simulink model "Senorless"  (R2023a)
settings: Solver=FixedStepDiscrete  StartTime=0.0  StopTime=5  FixedStep=1/FOC_FRQ  RelTol=1e-3
values from neighbouring files (symbols this model uses):
  ADC_REF = 3.6    [Senorless.sldd]
  ADC_SAMPLE_MAX = 32767.0    [Senorless.sldd]
  AMP_GAIN = 16.0    [Senorless.sldd]
  CURR_INPUT = 3276.0    [Senorless.sldd]
  CURR_KI = 380.0    [Senorless.sldd]
  CURR_KP = 0.04    [Senorless.sldd]
  CURR_LIMIT = 0.95    [Senorless.sldd]
  CURR_OVER = 6.0    [Senorless.sldd]
  CURR_POINT_GAIN = 7.0    [Senorless.sldd]
  CURR_STEP = 32760.0    [Senorless.sldd]
  CURR_UNDER = 0.03    [Senorless.sldd]
  CURR_WIDTH = 6552.0    [Senorless.sldd]
  FOC_FRQ = 25000.0    [Senorless.sldd]
  GAMMA = 32767.0    [Senorless.sldd]
  IMAX = 10.0    [Senorless.sldd]
  LPF_FRQ = 2000.0    [Senorless.sldd]
  MOTOR_DAMPER = 2.06E-7    [Senorless.sldd]
  MOTOR_FLUX = 0.00212352    [Senorless.sldd]
  MOTOR_INERTIA = 4.0E-7    [Senorless.sldd]
  MOTOR_LS = 0.000536    [Senorless.sldd]
  MOTOR_PN = 7.0    [Senorless.sldd]
  MOTOR_RS = 4.0    [Senorless.sldd]
  OPEN_IQ = 0.28    [Senorless.sldd]
  OPEN_IQ_MIN = 0.05    [Senorless.sldd]
  OPEN_IQ_SLOW = 0.1    [Senorless.sldd]
  OPEN_SPD = 1000.0    [Senorless.sldd]
  OPEN_SPD_SLOW = 180.0    [Senorless.sldd]
  OPEN_TIME = 0.5    [Senorless.sldd]
  OPEN_TIME_NFO = 0.5    [Senorless.sldd]
  PLL_LIMIT = 0.9    [Senorless.sldd]
  PLL_WIDTH = 800.0    [Senorless.sldd]
  PWM_FRQ = 96000000.0    [Senorless.sldd]
  RS_HUNT = 0.02    [Senorless.sldd]
  SMOK_FRQ = 600.0    [Senorless.sldd]
  SPD_LIMIT = 0.9    [Senorless.sldd]
  SPD_LPF_LEVEL = 0.0    [Senorless.sldd]
  SPD_MAX = 12000.0    [Senorless.sldd]
  SPD_MIN = 4000.0    [Senorless.sldd]
  SPD_REDUCE = 380.0    [Senorless.sldd]
  SPD_STEP = 6.0    [Senorless.sldd]
  SPD_WIDTH = 20.0    [Senorless.sldd]
  THETA_ERR_LIMIT = 8192.0    [Senorless.sldd]
  TS_POINT_GAIN = 10.0    [Senorless.sldd]
  UDC = 48.0    [Senorless.sldd]
  UDC_GAIN = 21.0    [Senorless.sldd]
  UDC_POINT_GAIN = 10.0    [Senorless.sldd]
undefined symbols (not defined in the file or in its folder): curr_q_ki, curr_q_kp, DiscIntNeverNeededParam, magnitude, PLL_LPF_LEVEL, Udc
libraries: simulink x20, slpidlib x5, mcbcontrolslib x2, mcbplantlib x1, autolibpmsmexterior x1, spspowerguiLib x1
(part 1 of 8)
settings Model: DataDictionary=Senorless.sldd  NumberOfSteps=100  SnapshotBufferSize=5000  SnapshotInterval=5000  Creator=lzm  LastModifiedBy=liangzhuoming
settings DataIOCC: ReturnWorkspaceOutputs=off
settings OptimizationCC: DefaultParameterBehavior=Inlined  GainParamInheritBuiltInType=on  UseFloatMulNetSlope=on  InheritOutputTypeSmallerThanSingle=on  DefaultUnderspecifiedDataType=single  UseSpecifiedMinMax=on  InlineInvariantSignals=on  PassReuseOutputArgsAs=Individual arguments  ZeroExternalMemoryAtStartup=off  ZeroInternalMemoryAtStartup=off  NoFixptDivByZeroProtection=on  EfficientFloat2IntCast=on  LifeSpan=1  OptimizeBlockOrder=speed  DifferentSizesBufferReuse=on  EfficientTunableParamExpr=on
settings DebuggingCC: SignalRangeChecking=warning  ParameterTunabilityLossMsg=error  UnconnectedInputMsg=warning  UnconnectedOutputMsg=warning  UnconnectedLineMsg=warning
settings HardwareCC: ProdBitPerPointer=32  ProdBitPerSizeT=32  ProdBitPerPtrDiffT=32  ProdLargestAtomicInteger=Long  ProdLargestAtomicFloat=Double  ProdWordSize=32  ProdLongLongMode=on  ProdHWDeviceType=ARM Compatible->ARM Cortex-M
settings ModelReferenceCC: EnableRefExpFcnMdlSchedulingChecks=on
settings SFSimCC: MATLABDynamicMemAlloc=off
settings RTWCC: Description=Embedded Coder  SystemTargetFile=ert.tlc  GenCodeOnly=on  TemplateMakefile=ert_default_tmf  GenerateReport=on  BuildConfiguration=Faster Runs  LaunchReport=on  GenerateCodeReplacementReport=on  DLArmComputeVersion=19.05
settings CodeAppCC: ForceParamTrailComments=on  IgnoreCustomStorageClasses=off  OperatorAnnotations=on  SimulinkDataObjDesc=on  SFDataObjDesc=on  CustomSymbolStrGlobalVar=rt$N$M  CustomSymbolStrType=$N$M  CustomSymbolStrFcn=$N$M$F  CustomSymbolStrMacro=$N$M  InsertBlockDesc=on
settings ERTTargetCC: TargetLangStandard=C99 (ISO)  GenerateSampleERTMain=on  IncludeMdlTerminateFcn=off  CombineSignalStateStructs=on  SupportNonFinite=off  SupportComplex=off  SupportNonInlinedSFcns=on  InlinedParameterPlacement=NonHierarchical  ERTCustomFileTemplate=example_file_process.tlc  ERTFilePackagingFormat=CompactWithDataFile

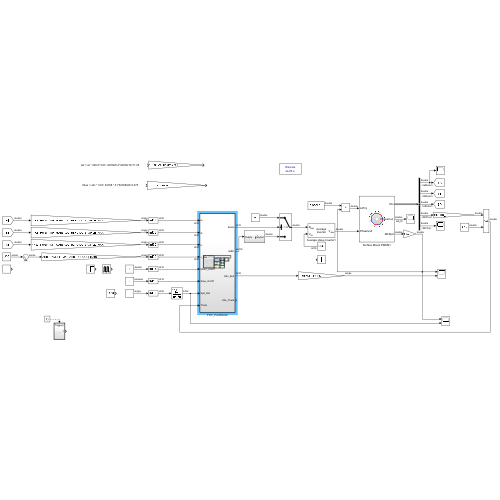
[thumbnail: Simulink's stored preview of the top-level diagram]
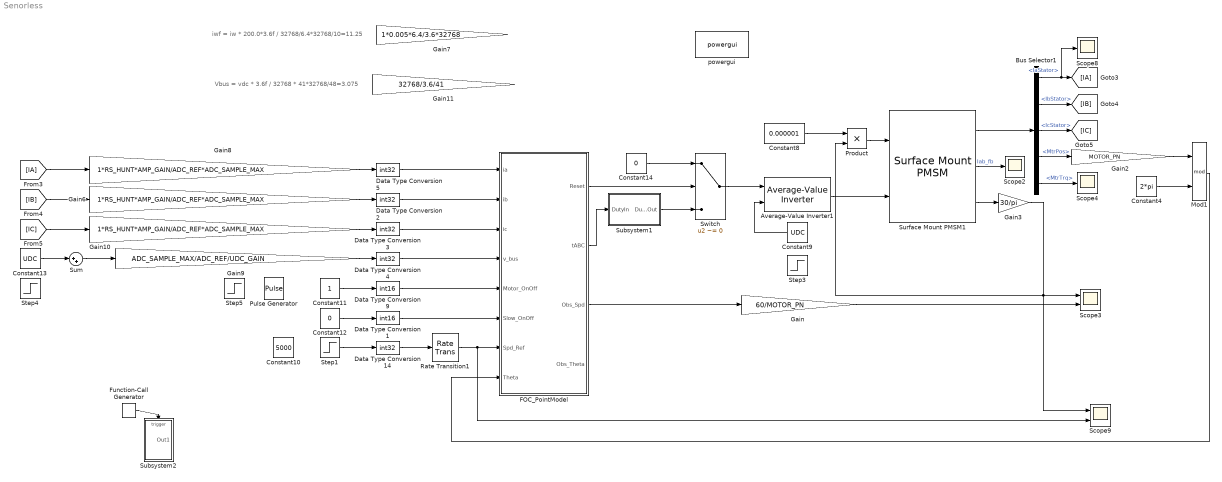
== system Senorless ==
  note: iwf = iw * 200.0*3.6f / 32768/6.4*32768/10=11.25
  note: Vbus = vdc * 3.6f / 32768 * 41*32768/48=3.075
  Average-Value Inverter1 : mcbplantlib/Average-Value Inverter
  Bus Selector1 : BusSelector  OutputSignals=IaStator,IbStator,IcStator,MtrPos,MtrTrq
  Constant10 : Constant  Value=5000  OutDataTypeStr=int16
  Constant11 : Constant
  Constant12 : Constant  Value=0  OutDataTypeStr=boolean
  Constant13 : Constant  Value=UDC  OutDataTypeStr=single
  Constant14 : Constant  Value=0
  Constant4 : Constant  Value=2*pi
  Constant8 : Constant  Value=0.000001
  Constant9 : Constant  Value=UDC
  Data Type Conversion1 : DataTypeConversion  OutDataTypeStr=int16  SaturateOnIntegerOverflow=off  RndMeth=Floor
  Data Type Conversion{2..5,14} (5 alike) : DataTypeConversion  OutDataTypeStr=int32  SaturateOnIntegerOverflow=off  RndMeth=Floor
  Data Type Conversion9 : DataTypeConversion  OutDataTypeStr=int16  SaturateOnIntegerOverflow=off  RndMeth=Floor
  FOC_PointModel : Subsystem  TreatAsAtomicUnit=on
      settings: RTWSystemCode=Nonreusable function
  Function-Call Generator : simulink/Ports & Subsystems/Function-Call Generator  sample_time=1/2500*10  numberOfIterations=1  DisallowWideOutput=off
  Gain : Gain  Gain=60/MOTOR_PN  OutDataTypeStr=single  RndMeth=Zero
  Gain10 : Gain  Gain=1*RS_HUNT*AMP_GAIN/ADC_REF*ADC_SAMPLE_MAX  OutDataTypeStr=single
  Gain11 : Gain  Gain=32768/3.6/41
  Gain2 : Gain  Gain=MOTOR_PN
  Gain3 : Gain  Gain=30/pi
  Gain6 : Gain  Gain=1*RS_HUNT*AMP_GAIN/ADC_REF*ADC_SAMPLE_MAX  OutDataTypeStr=single
  Gain7 : Gain  Gain=1*0.005*6.4/3.6*32768
  Gain8 : Gain  Gain=1*RS_HUNT*AMP_GAIN/ADC_REF*ADC_SAMPLE_MAX  OutDataTypeStr=single
  Gain9 : Gain  Gain=ADC_SAMPLE_MAX/ADC_REF/UDC_GAIN
  Mod1 : Math  Operator=mod
  Product : Product
  Pulse Generator : DiscretePulseGenerator  PulseType=Time based  Period=2.2  PulseWidth=99
  Rate Transition1 : RateTransition
  Scope2 : Scope
  Scope3 : Scope  NumInputPorts=2
  Scope4 : Scope
  Scope8 : Scope
  Scope9 : Scope  NumInputPorts=2
  Step1 : Step  Time=2.5  Before=32000  After=2000  OutDataTypeStr=single  SampleTime=0
  Step3 : Step  Time=2.5  Before=48  After=47  OutDataTypeStr=single  SampleTime=0
  Step4 : Step  Time=2.5  Before=48  After=47  OutDataTypeStr=single  SampleTime=0
  Step5 : Step  Time=3  SampleTime=0
  Subsystem1 : Subsystem
  Subsystem2 : Subsystem
  Sum : Sum  Inputs=|++
  Surface Mount PMSM1 : autolibpmsmexterior/Surface Mount PMSM  port_config=Torque  sim_type=Discrete  Ts=1/FOC_FRQ  P=MOTOR_PN  Rs=MOTOR_RS  Ldq_=MOTOR_LS  KConstText=Permanent flux linkage constant (lambda_pm):  lambda_pm=MOTOR_FLUX  Ke=0.0059268  Kt=0.061  mechanical=[MOTOR_INERTIA, MOTOR_DAMPER, 0]  idq0=[0 0]  theta_init=4/5  omega_init=0  KConst=MOTOR_FLUX  lambda_pm_calc=MOTOR_FLUX  RefBlkName='autolibpmsmexterior/Surface Mount PMSM'  aMode=5  Ldq="[0.0017      0.0017]"
  Switch : Switch  Criteria=u2 ~= 0  SaturateOnIntegerOverflow=off  InputSameDT=off
  powergui : spspowerguiLib/powergui  Priority=1  SimulationMode=Discrete  SampleTime=1/25000  frequency=60  Iterations=50  frequencyindice=60  Pbase=100e6  ErrMax=1e-4  UnitsV=kV  UnitsW=MW  buscounter=0  FunctionMessages=off  echomessages=off  EnableUseOfTLC=off  CurrentSourceSwitches=off  DisableSnubberDevices=off  DisableRonSwitches=off  DisableVfSwitches=off  DisplayEquations=off  AutomaticDiscreteSolvers=off  SolverType=Tustin/Backward Euler (TBE)  Interpol=off  ExternalGateDelay=off  methode=off  Ts=100  x0status=blocks  SPID=on  SwTol=0  HookPort=off  NonlinearTolerance=1e-4  nMaxIteration=100  ContinueOnMaxIteration=off  RestoreLinks=warning  ResistiveCurrentMeasurement=off  Frange=[0:2:500]  Ylog=off  Xlog=on  ShowGrid=off  save=off  variable=ZData  structure=0  ZoomFFT=off  StartTime=0.0  cycles=1  DisplayStyle=1  fundamental=60  FreqAxis=off  MaxFrequency=1000  frequencyindicesteady=1  RmsSteady=1  display=off
  wires:
  Surface Mount PMSM1/3 -> Gain3/1
  Surface Mount PMSM1/2 -> Scope2/1  "Iab_fb"
  Surface Mount PMSM1/1 -> Bus Selector1/1
  Bus Selector1/1 -> Scope8/1, [IA]  "<IaStator>"
  Bus Selector1/2 -> [IB]  "<IbStator>"
  Bus Selector1/3 -> [IC]  "<IcStator>"
  Constant4/1 -> Mod1/2
  Gain2/1 -> Mod1/1
  Bus Selector1/4 -> Gain2/1  "<MtrPos>"
  Data Type Conversion5/1 -> FOC_PointModel/1(ia)
  Data Type Conversion2/1 -> FOC_PointModel/2(ib)
  Data Type Conversion3/1 -> FOC_PointModel/3(ic)
  Data Type Conversion9/1 -> FOC_PointModel/5(Motor_OnOff)
  [IC] -> Gain10/1
  Gain8/1 -> Data Type Conversion5/1
  Gain6/1 -> Data Type Conversion2/1
  Gain10/1 -> Data Type Conversion3/1
  Gain9/1 -> Data Type Conversion4/1
  [IB] -> Gain6/1
  [IA] -> Gain8/1
  FOC_PointModel/2(tABC) -> Subsystem1/1(DutyIn)
  Gain3/1 -> Scope9/1, Scope3/1, Product/2
  Sum/1 -> Gain9/1
  Data Type Conversion4/1 -> FOC_PointModel/4(v_bus)
  FOC_PointModel/3(Obs_Spd) -> Gain/1
  Mod1/1 -> FOC_PointModel/8(Theta)
  Gain/1 -> Scope3/2
  Data Type Conversion14/1 -> Rate Transition1/1
  Constant8/1 -> Product/1
  Data Type Conversion1/1 -> FOC_PointModel/6(Slow_OnOff)
  Constant12/1 -> Data Type Conversion1/1
  Subsystem1/1(DutyOut) -> Switch/3
  Bus Selector1/5 -> Scope4/1  "<MtrTrq>"
  Average-Value Inverter1/1 -> Surface Mount PMSM1/2
  Switch/1 -> Average-Value Inverter1/1
  FOC_PointModel/1(Reset) -> Switch/2
  Constant14/1 -> Switch/1
  Constant9/1 -> Average-Value Inverter1/2
  Constant13/1 -> Sum/1
  Product/1 -> Surface Mount PMSM1/1
  Rate Transition1/1 -> Scope9/2, FOC_PointModel/7(Spd_Ref)
  Function-Call Generator/1 -> Subsystem2/Trigger
  Step1/1 -> Data Type Conversion14/1
  Constant11/1 -> Data Type Conversion9/1

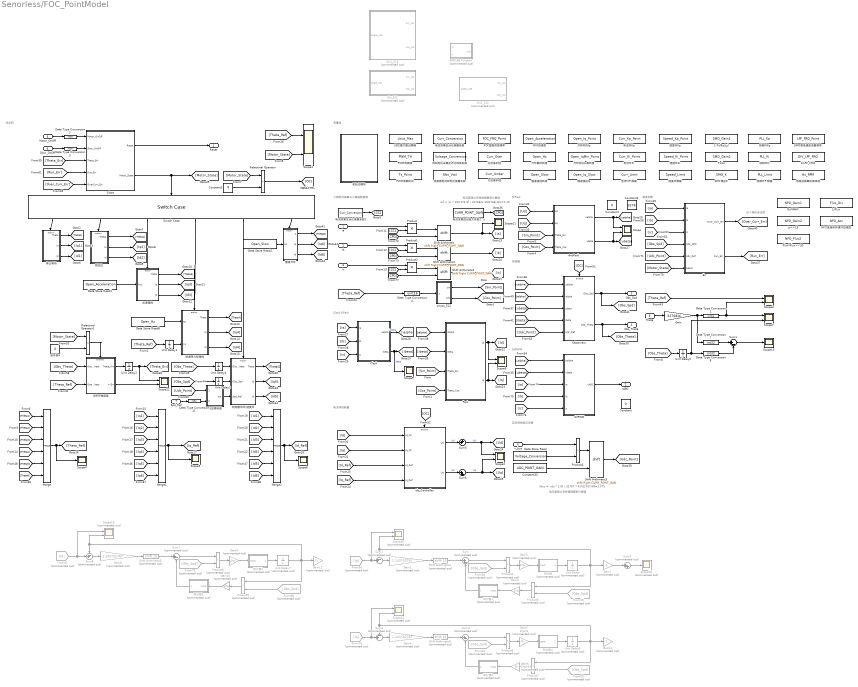
== system Senorless/FOC_PointModel ==
  note: 这个用在全过程
  note: 错误判断
  note: 观测器
  note: SVPWM
  note: 反Park
  note: 实时母线电压采集
  note: 电流环控制器
  note: Clark与Park
  note: 三相电流换算与三角函数查表
  note: 变量池
  note: 状态机
  note: 电流直接从采样值换算到计算值
  note: Vbus = vdc * 3.6f / 32767 * 41*32767/48=3.075
  note: iwf = iw * 200.0*3.6f / 32768/6.4*32768/10=11.25
  note: 电压直接从采样值换算到计算值
  ia : Inport  OutDataTypeStr=int32
  ib : Inport  Port=2  OutDataTypeStr=int32
  ic : Inport  Port=3  OutDataTypeStr=int32
  v_bus : Inport  Port=4  OutDataTypeStr=int32
  Motor_OnOff : Inport  Port=5
  Slow_OnOff : Inport  Port=6
  Spd_Ref : Inport  Port=7
  Theta : Inport  Port=8
  1-Ts(Rs/Ls) : DataStoreMemory  DataStoreName=SMO_Gain1  WriteAfterWriteMsg=warning  ShowAdditionalParam=off
  1/Flux : DataStoreMemory  DataStoreName=Flux_Div  WriteAfterWriteMsg=warning  ShowAdditionalParam=off
  1/LPF_FRQ : DataStoreMemory  DataStoreName=DIV_LPF_FRQ  WriteAfterWriteMsg=warning  ShowAdditionalParam=off
  AntiPark : Subsystem
  Chart : Stateflow chart  TreatAsAtomicUnit=on
  Clark : Subsystem
  Constant : Constant  Value=0  OutDataTypeStr=uint16
  Constant1 : Constant  Value=0  OutDataTypeStr=int16
  Constant2 : Constant  Value=3276  OutDataTypeStr=int16
  Constant3 : Constant  Value=0  OutDataTypeStr=uint8
  Constant33 : Constant  Value=UDC_POINT_GAIN
  Data Store Read : DataStoreRead  DataStoreName=Voltage_Conversion  IndexOptions=Index vector (dialog)  Indices=1  OutputSizes=1
  Data Store Read1 : DataStoreRead  DataStoreName=Open_Acceleration  IndexOptions=Index vector (dialog)  Indices=1  OutputSizes=1
  Data Store Read2 : DataStoreRead  DataStoreName=Open_Slow  IndexOptions=Index vector (dialog)  Indices=1  OutputSizes=1
  Data Store Read6 : DataStoreRead  DataStoreName=Open_Hz  IndexOptions=Index vector (dialog)  Indices=1  OutputSizes=1
  Data Type Conversion1 : DataTypeConversion  OutDataTypeStr=uint16  SaturateOnIntegerOverflow=off  RndMeth=Floor
  Data Type Conversion11 : DataTypeConversion  OutDataTypeStr=int32  SaturateOnIntegerOverflow=off
  Data Type Conversion2 : DataTypeConversion  OutDataTypeStr=int16  SaturateOnIntegerOverflow=off
  Data Type Conversion3 : DataTypeConversion  OutDataTypeStr=int16  SaturateOnIntegerOverflow=off
  Data Type Conversion4 : DataTypeConversion  OutDataTypeStr=uint16  SaturateOnIntegerOverflow=off
  Data Type Conversion7 : DataTypeConversion  OutDataTypeStr=int32  SaturateOnIntegerOverflow=off
  Data Type Conversion8 : DataTypeConversion  OutDataTypeStr=int32  SaturateOnIntegerOverflow=off
  Err : Subsystem
  FOC整数类型频率 : DataStoreMemory  DataStoreName=FOC_FRQ_Point  WriteAfterWriteMsg=warning  ShowAdditionalParam=off
  Flux*Flux<<30 : DataStoreMemory  DataStoreName=NFO_Flux2  WriteAfterWriteMsg=warning  ShowAdditionalParam=off
  From{54..55,62,69,79..80} (6 alike) : From  Commented=on  GotoTag=Obs_Spd
  From56 : From  Commented=on  GotoTag=Iq
  From78 : From  Commented=on  GotoTag=Iq
  From81 : From  Commented=on  GotoTag=Id
  Gain : Gain  Gain=32768/pi
  Gain1 : Gain  Commented=on  Gain=1.141*32767  ParamDataTypeStr=int32  OutDataTypeStr=int32  RndMeth=Zero
  Gain{2..3,9..10} (4 alike) : Gain  Commented=on  Gain=2*pi  ParamDataTypeStr=int16  OutDataTypeStr=int32  RndMeth=Zero
  Gain11 : Gain  Commented=on  Gain=-1  ParamDataTypeStr=int16  OutDataTypeStr=int32
  Gain12 : Gain  Commented=on  Gain=-1  ParamDataTypeStr=int16  OutDataTypeStr=int32
  Gain4 : Gain  Commented=on  Gain=1.141*32767  ParamDataTypeStr=int32  OutDataTypeStr=int32  RndMeth=Zero
  Gain5 : Gain  Commented=on  Gain=2*pi*3  ParamDataTypeStr=int16  OutDataTypeStr=int32  RndMeth=Zero
  Gain6 : Gain  Commented=on  Gain=2*pi*3  ParamDataTypeStr=int16  OutDataTypeStr=int32  RndMeth=Zero
  Gain7 : Gain  Commented=on  Gain=-2  ParamDataTypeStr=int16  OutDataTypeStr=int32
  Gain8 : Gain  Commented=on  Gain=1.141*32767  ParamDataTypeStr=int32  OutDataTypeStr=int32  RndMeth=Zero
  Ls<<15 : DataStoreMemory  DataStoreName=NFO_Gain2  WriteAfterWriteMsg=warning  ShowAdditionalParam=off
  MATLAB Function : MATLAB Function  Commented=on  TreatAsAtomicUnit=on
  Merge : Merge  Inputs=6
  Merge1 : Merge  Inputs=6
  Merge2 : Merge  Inputs=6
  NFO直接闭环缓冲加速度 : DataStoreMemory  DataStoreName=NFO_Acc  WriteAfterWriteMsg=warning  ShowAdditionalParam=off
  Observers : Subsystem
  PWM周期值 : DataStoreMemory  DataStoreName=PWM_TH  WriteAfterWriteMsg=warning  ShowAdditionalParam=off
  PWM周期时间 : DataStoreMemory  DataStoreName=Ts_Point  WriteAfterWriteMsg=warning  ShowAdditionalParam=off
  Park : Subsystem
  Product{,1..3} (4 alike) : Product  OutDataTypeStr=int32  RndMeth=Zero
  Product{4..9} (6 alike) : Product  Commented=on  OutDataTypeStr=int32
  Relational Operator : RelationalOperator  Operator=>  OutDataTypeStr=boolean  RndMeth=Zero  InputSameDT=off
  Relational Operator1 : RelationalOperator  Operator=<  OutDataTypeStr=boolean  RndMeth=Zero  InputSameDT=off
  Rs*IMAX : DataStoreMemory  DataStoreName=NFO_Gain1  WriteAfterWriteMsg=warning  ShowAdditionalParam=off
  SMO增益K : DataStoreMemory  DataStoreName=SMO_K  WriteAfterWriteMsg=warning  ShowAdditionalParam=off
  SMO里低通滤波器频率 : DataStoreMemory  DataStoreName=LPF_FRQ_Point  WriteAfterWriteMsg=warning  ShowAdditionalParam=off
  SVPWM : Subsystem  ScheduleAs=Aperiodic partition  PartitionName=TEMP_PRECOMP_PARTITION_NAME_MessageTriggeredSubsystem
  Scope{,1..3,7..8,12} (7 alike) : Scope  NumInputPorts=2
  Scope10 : Scope  Commented=on  NumInputPorts=2
  Scope{4..6,9,11,13} (6 alike) : Scope
  Scope14 : Scope  Commented=on  NumInputPorts=2
  Scope15 : Scope  Commented=on
  Scope19 : Scope  Commented=on  NumInputPorts=2
  Shift Arithmetic{,1..3} (4 alike) : ArithShift  BitShiftNumberSource=Input port  BitShiftNumber=CURR_POINT_GAIN  BitShiftDirection=Right
      settings: InputPortMap=u0,p1
  Shift Arithmetic4 : ArithShift  Commented=on  BitShiftNumber=15
  Shift Arithmetic5 : ArithShift  Commented=on  BitShiftNumber=15
  Shift Arithmetic6 : ArithShift  Commented=on  BitShiftNumber=15
  Sin1_512 : MATLAB Function  Commented=on  TreatAsAtomicUnit=on
  Sin2_512 : MATLAB Function  Commented=on  TreatAsAtomicUnit=on
  Sin_512 : MATLAB Function  Commented=on  TreatAsAtomicUnit=on
  Sum : Sum  Commented=on  Inputs=|+-
  Sum1 : Sum  Inputs=|+-  OutDataTypeStr=int32
  Sum2 : Sum  Commented=on  Inputs=-+|
  Sum3 : Sum  Commented=on  Inputs=|+-
  Sum4 : Sum  Commented=on  Inputs=-+|
  Sum5 : Sum  Inputs=++|
  Sum6 : Sum  Inputs=|++
  Sum7 : Sum  Commented=on  Inputs=|+-
  Sum8 : Sum  Commented=on  Inputs=-+|
  Sum9 : Sum  Commented=on  Inputs=|++
  Switch Case : SwitchCase  CaseConditions={0,1,2,3,4,5}  ShowDefaultCase=off
  Ts/Ls : DataStoreMemory  DataStoreName=SMO_Gain2  WriteAfterWriteMsg=warning  ShowAdditionalParam=off
  UDQ最大输出限幅 : DataStoreMemory  DataStoreName=Uout_Max  WriteAfterWriteMsg=warning  ShowAdditionalParam=off
  Unit Delay : UnitDelay  Commented=on  SampleTime=-1  HasFrameUpgradeWarning=on
  Unit Delay{1..5} (5 alike) : UnitDelay  SampleTime=-1  HasFrameUpgradeWarning=on
  Unit Delay6 : UnitDelay  Commented=on  SampleTime=-1  HasFrameUpgradeWarning=on
  Unit Delay7 : UnitDelay  Commented=on  SampleTime=-1  HasFrameUpgradeWarning=on
  idq_Controller : Subsystem
  sincos_512 : Subsystem
  停止等待 : Subsystem  TreatAsAtomicUnit=on
  切闭环角度差 : Subsystem
  初始化模块 : Subsystem  TreatAsAtomicUnit=on
  加速强拖 : Subsystem  TreatAsAtomicUnit=on
  开环加速度 : DataStoreMemory  DataStoreName=Open_Acceleration  WriteAfterWriteMsg=warning  ShowAdditionalParam=off
  开环最终转速 : DataStoreMemory  DataStoreName=Open_Hz  WriteAfterWriteMsg=warning  ShowAdditionalParam=off
  开环阶段Iq : DataStoreMemory  DataStoreName=Open_Iq_Point  WriteAfterWriteMsg=warning  ShowAdditionalParam=off
  开环阶段Iq最终值 : DataStoreMemory  DataStoreName=Open_IqMin_Point  WriteAfterWriteMsg=warning  ShowAdditionalParam=off
  恒速降力矩强拖 : Subsystem  TreatAsAtomicUnit=on
  慢速开环 : Subsystem  TreatAsAtomicUnit=on
  慢速强拖Iq : DataStoreMemory  DataStoreName=Open_Iq_Slow  WriteAfterWriteMsg=warning  ShowAdditionalParam=off
  慢速强拖转速 : DataStoreMemory  DataStoreName=Open_Slow  WriteAfterWriteMsg=warning  ShowAdditionalParam=off
  欠流保护值 : DataStoreMemory  DataStoreName=Curr_Under  WriteAfterWriteMsg=warning  ShowAdditionalParam=off
  母线电压采集定点化转换系数 : DataStoreMemory  DataStoreName=Voltage_Conversion  WriteAfterWriteMsg=warning  ShowAdditionalParam=off
  电压限转速 : Subsystem
  电流环Ki : DataStoreMemory  DataStoreName=Curr_Ki_Point  WriteAfterWriteMsg=warning  ShowAdditionalParam=off
  电流环Kp : DataStoreMemory  DataStoreName=Curr_Kp_Point  WriteAfterWriteMsg=warning  ShowAdditionalParam=off
  电流环PI限幅 : DataStoreMemory  DataStoreName=Curr_Limit  WriteAfterWriteMsg=warning  ShowAdditionalParam=off
  电流采集定点化换算系数 : DataStoreMemory  DataStoreName=Curr_Conversion  WriteAfterWriteMsg=warning  ShowAdditionalParam=off
  电流采集定点化换算系数1 : DataStoreRead  DataStoreName=Curr_Conversion  IndexOptions=Index vector (dialog)  Indices=1  OutputSizes=1
  电流采集适当放大系数2^n : Constant  Value=CURR_POINT_GAIN
  电赫兹换算机械转速 : DataStoreMemory  DataStoreName=Hz_RPM  WriteAfterWriteMsg=warning  ShowAdditionalParam=off
  积分器 : Subsystem  Commented=on
      settings: MinAlgLoopOccurrences=on
  积分器1 : Subsystem  Commented=on
      settings: MinAlgLoopOccurrences=on
  积分器2 : Subsystem  Commented=on
      settings: MinAlgLoopOccurrences=on
  积分器3 : Subsystem  Commented=on
      settings: MinAlgLoopOccurrences=on
  积分器4 : Subsystem  Commented=on
      settings: MinAlgLoopOccurrences=on
  积分器5 : Subsystem  Commented=on
      settings: MinAlgLoopOccurrences=on
  观测器电流转电压衡量系数 : DataStoreMemory  DataStoreName=Obs_VtoI  WriteAfterWriteMsg=warning  ShowAdditionalParam=off
  观测器闭环/速度环 : Subsystem  TreatAsAtomicUnit=on
  过流保护值 : DataStoreMemory  DataStoreName=Curr_Over  WriteAfterWriteMsg=warning  ShowAdditionalParam=off
  速度环Ki : DataStoreMemory  DataStoreName=Speed_Ki_Point  WriteAfterWriteMsg=warning  ShowAdditionalParam=off
  速度环Kp : DataStoreMemory  DataStoreName=Speed_Kp_Point  WriteAfterWriteMsg=warning  ShowAdditionalParam=off
  速度环限幅 : DataStoreMemory  DataStoreName=Speed_Limit  WriteAfterWriteMsg=warning  ShowAdditionalParam=off
  锁相环Ki : DataStoreMemory  DataStoreName=PLL_Ki  WriteAfterWriteMsg=warning  ShowAdditionalParam=off
  锁相环Kp : DataStoreMemory  DataStoreName=PLL_Kp  WriteAfterWriteMsg=warning  ShowAdditionalParam=off
  锁相环PI限幅 : DataStoreMemory  DataStoreName=PLL_Limit  WriteAfterWriteMsg=warning  ShowAdditionalParam=off
  闭环是4 : Constant  Value=4  OutDataTypeStr=uint8
  预定位 : Subsystem  TreatAsAtomicUnit=on
  Reset : Outport
  tABC : Outport  Port=2
  Obs_Spd : Outport  Port=3
  Obs_Theta : Outport  Port=4
  wires:
  Motor_OnOff/1 -> Data Type Conversion2/1
  Switch Case/1 -> 停止等待/Action
  Switch Case/3 -> 加速强拖/Action
  Switch Case/2 -> 预定位/Action
  Switch Case/4 -> 恒速降力矩强拖/Action
  [Sin_Point] -> AntiPark/3(Theta_Sin)
  [Cos_Point] -> AntiPark/4(Theta_Cos)
  v_bus/1 -> Product3/1
  Product1/1 -> Shift Arithmetic1/1
  Product2/1 -> Shift Arithmetic2/1
  电流采集定点化换算系数1/1 -> [CC]
  [CC] -> Product/2
  [CC] -> Product1/2
  Data Store Read/1 -> Product3/2
  Unit Delay1/1 -> 恒速降力矩强拖/2(Xo)
  Data Store Read6/1 -> 恒速降力矩强拖/1(Hz)
  Data Store Read1/1 -> 加速强拖/1(Acc)
  停止等待/1(Theta) -> [Theta1]
  停止等待/2(Iq) -> [Iq1]
  停止等待/3(Id) -> [Id1]
  预定位/1(Theta) -> [Theta2]
  预定位/2(Iq) -> [Iq2]
  预定位/3(Id) -> [Id2]
  加速强拖/1(Theta) -> [Theta3]
  加速强拖/2(Iq) -> [Iq3]
  加速强拖/3(Id) -> [Id3]
  恒速降力矩强拖/2(Iq) -> [Iq4]
  恒速降力矩强拖/3(Id) -> [Id4]
  [Theta_Ref] -> Unit Delay1/1
  [Theta1] -> Merge/1
  [Theta2] -> Merge/2
  [Theta3] -> Merge/3
  [Theta4] -> Merge/4
  [Iq1] -> Merge1/1
  [Iq2] -> Merge1/2
  [Iq3] -> Merge1/3
  [Iq4] -> Merge1/4
  Merge1/1 -> [Iq_Ref], Scope5/1
  [Id1] -> Merge2/1
  [Id2] -> Merge2/2
  [Id3] -> Merge2/3
  [Id4] -> Merge2/4
  Merge2/1 -> [Id_Ref], Scope6/1
  [Id_Ref] -> idq_Controller/3(Id_Ref)
  [Iq_Ref] -> idq_Controller/4(Iq_Ref)
  Shift Arithmetic/1 -> Scope11/1, [ia]
  Shift Arithmetic1/1 -> [ib]
  Shift Arithmetic2/1 -> [ic]
  [ia] -> Clark/1(ia)
  [ib] -> Clark/2(ib)
  [ic] -> Clark/3(ic)
  [Iq] -> idq_Controller/2(Iq_Fd)
  [Id] -> idq_Controller/1(Id_Fd)
  [ualpha] -> SVPWM/1(Ualpha)
  [ubeta] -> SVPWM/2(Ubeta)
  Clark/1(ialpha) -> [ialpha]  "ialpha"
  Clark/2(ibeta) -> Scope9/1, [ibeta]  "ibeta"
  [ualpha] -> Observers/1(ualpha)
  [ibeta] -> Observers/4(ibeta)
  [ubeta] -> Observers/3(ubeta)
  [ialpha] -> Observers/2(ialpha)
  Observers/1(Obs_Spd) -> Obs_Spd/1, [Obs_Spd]
  恒速降力矩强拖/1(Theta) -> [Theta4]
  Observers/2(Obs_Theta) -> Obs_Theta/1, [Obs_Theta]
  Switch Case/5 -> 观测器闭环/速度环/Action
  观测器闭环/速度环/1(Theta) -> [Theta5]
  观测器闭环/速度环/2(Iq) -> [Iq5]
  观测器闭环/速度环/3(Id) -> [Id5]
  [Iq5] -> Merge1/5
  [Id5] -> Merge2/5
  Data Type Conversion4/1 -> sincos_512/1(theta)
  Theta/1 -> Gain/1
  [Theta5] -> Merge/5
  Gain/1 -> Data Type Conversion7/1, Data Type Conversion1/1
  [Theta_Ref] -> Data Type Conversion4/1
  sincos_512/2(cos) -> [Cos_Point]
  Data Type Conversion1/1 -> Scope7/1, Scope3/2
  [Theta_Ref] -> Scope1/1
  Chart/2(Motor_State) -> Switch Case/1, [Motor_State]
  Merge/1 -> Scope4/1, [Theta_Ref]
  Sum1/1 -> Scope13/1
  Data Type Conversion7/1 -> Sum1/1
  Data Type Conversion8/1 -> Sum1/2
  [Obs_Theta] -> Unit Delay4/1
  [Obs_Theta] -> Unit Delay5/1
  [CC] -> Product2/2
  Product3/1 -> Shift Arithmetic3/1
  Constant33/1 -> Shift Arithmetic3/2
  [Theta_Err] -> Chart/3(Theta_Err)
  [Theta_Ref] -> Scope3/1
  [Obs_Spd] -> Unit Delay3/1
  [Run_Err] -> Chart/4(Run_Err)
  SVPWM/1(tABC) -> tABC/1
  Chart/1(Reset) -> Reset/1
  Unit Delay4/1 -> 观测器闭环/速度环/1(Obs_Theta)
  Unit Delay3/1 -> 观测器闭环/速度环/2(Obs_Spd)
  Shift Arithmetic3/1 -> [Udc_Point]
  电压限转速/1(out) -> 观测器闭环/速度环/3(Spd_Ref)
  Spd_Ref/1 -> Data Type Conversion11/1
  [Udc_Point] -> 电压限转速/1(Udc_Ref)
  [Over_Curr_Err] -> Chart/5(OverCurr_Err)
  Slow_OnOff/1 -> Data Type Conversion3/1
  Data Type Conversion3/1 -> Chart/2(Slow_OnOff)
  ia/1 -> Product/1
  ib/1 -> Product1/1
  ic/1 -> Product2/1
  Data Type Conversion11/1 -> 电压限转速/2(SPD_Ref)
  Data Type Conversion2/1 -> Chart/1(Motor_OnOff)
  Switch Case/6 -> 慢速开环/Action
  慢速开环/1(Theta) -> [Theta6]
  慢速开环/2(Iq) -> [Iq6]
  慢速开环/3(Id) -> [Id6]
  [Theta6] -> Merge/6
  [Iq6] -> Merge1/6
  [Id6] -> Merge2/6
  Sum5/1 -> [Ud], Scope2/1  "Ud"
  Sum6/1 -> [Uq], Scope2/2  "Uq"
  [ia] -> Err/1(ia)
  [ib] -> Err/2(ib)
  [ic] -> Err/3(ic)
  [Obs_Spd] -> Err/4(Obs_SPD)
  Err/1(Over_Curr_Err) -> [Over_Curr_Err]
  Err/2(Run_Err) -> [Run_Err]
  [Motor_State] -> Err/6(Reset)
  [Udc_Point] -> Observers/5(Udc_Ref)
  [Udc_Point] -> Err/5(Udc_Ref)
  AntiPark/1(ualpha) -> Scope/1, [ualpha]
  AntiPark/2(ubeta) -> Scope/2, [ubeta]
  [Ud] -> AntiPark/1(Ud)
  [Uq] -> AntiPark/2(Uq)
  [ia] -> SVPWM/3(ia)
  [ib] -> SVPWM/4(ib)
  [ic] -> SVPWM/5(ic)
  sincos_512/1(sin) -> [Sin_Point]
  [CPG] -> Shift Arithmetic/2
  [CPG] -> Shift Arithmetic1/2
  [CPG] -> Shift Arithmetic2/2
  Product/1 -> Shift Arithmetic/1
  电流采集适当放大系数2^n/1 -> [CPG]
  [Motor_State] -> Scope1/2
  Relational Operator/1 -> [OC]
  [Motor_State] -> Relational Operator/1
  Constant3/1 -> Relational Operator/2
  [OC] -> idq_Controller/Enable
  [OC] -> Observers/Enable
  切闭环角度差/1(Theta_Rrr) -> Unit Delay2/1
  [Obs_Theta] -> 切闭环角度差/1(Obs_Theta)
  [Theta_Ref] -> 切闭环角度差/2(Open_Theta)
  切闭环角度差/2(+-Err) -> Scope12/2
  闭环是4/1 -> Relational Operator1/2
  [Motor_State] -> Relational Operator1/1
  Relational Operator1/1 -> 切闭环角度差/Enable
  Unit Delay2/1 -> Scope12/1, [Theta_Err]
  Data Store Read2/1 -> 慢速开环/1(Hz)
  Park/1(Id) -> [Id], Scope8/1
  Park/2(Iq) -> [Iq], Scope8/2
  [ialpha] -> Park/1(ialpha)
  [ibeta] -> Park/2(ibeta)
  [Sin_Point] -> Park/3(Theta_Sin)
  [Cos_Point] -> Park/4(Theta_Cos)
  Unit Delay5/1 -> Data Type Conversion8/1, Scope7/2
  Sum2/1 -> Gain1/1
  Gain1/1 -> Shift Arithmetic4/1
  积分器/1(output) -> Unit Delay/1
  From54/1 -> Product4/2
  From55/1 -> Product5/2
  积分器1/1(output) -> Sum/2
  Sum/1 -> Product4/1
  Product5/1 -> Gain3/1
  Product4/1 -> Gain2/1
  From56/1 -> Scope10/1, Sum2/2
  Unit Delay/1 -> Gain7/1, Sum2/1, Scope10/2, Product5/1
  Gain2/1 -> 积分器/1(input)
  Gain3/1 -> 积分器1/1(input)
  Shift Arithmetic4/1 -> Sum/1
  idq_Controller/1(Ud) -> Sum5/2  "Ud"
  idq_Controller/2(Uq) -> Sum6/1  "Uq"
  Shift Arithmetic5/1 -> Sum7/1
  Gain10/1 -> 积分器3/1(input)
  Gain9/1 -> 积分器2/1(input)
  Unit Delay7/1 -> Product9/1, Scope19/2, Sum8/1, Gain11/1
  From81/1 -> Sum8/2, Scope19/1
  Product8/1 -> Gain9/1
  Product9/1 -> Gain10/1
  Sum7/1 -> Product8/1
  积分器3/1(output) -> Sum7/2
  From80/1 -> Product9/2
  From79/1 -> Product8/2
  积分器2/1(output) -> Unit Delay7/1
  Gain8/1 -> Shift Arithmetic5/1
  Sum8/1 -> Gain8/1
  Gain7/1 -> Sum9/1
  Sum9/1 -> Scope15/1
  Shift Arithmetic6/1 -> Sum3/1
  Gain6/1 -> 积分器5/1(input)
  Gain5/1 -> 积分器4/1(input)
  Unit Delay6/1 -> Product7/1, Scope14/2, Sum4/1, Gain12/1
  From78/1 -> Sum4/2, Scope14/1
  Product6/1 -> Gain5/1
  Product7/1 -> Gain6/1
  Sum3/1 -> Product6/1
  积分器5/1(output) -> Sum3/2
  From69/1 -> Product7/2
  From62/1 -> Product6/2
  积分器4/1(output) -> Unit Delay6/1
  Gain4/1 -> Shift Arithmetic6/1
  Sum4/1 -> Gain4/1

== system Senorless/Subsystem1 ==
  DutyIn : Inport
  Constant : Constant  Value=0.5  SampleTime=-1
  Constant1 : Constant  SampleTime=-1
  Constant2 : Constant  Value=0.5  SampleTime=-1
  Constant7 : Constant  Value=PWM_FRQ
  Constant8 : Constant  Value=FOC_FRQ*2
  Dead Zone : DeadZone  LowerValue=-10/(PWM_FRQ/FOC_FRQ/2)  UpperValue=10/(PWM_FRQ/FOC_FRQ/2)  SaturateOnIntegerOverflow=off
  Display : Display
  Divide : Product  Inputs=*/
  Divide2 : Product  Inputs=*/
  Gain1 : Gain  Gain=-1
  Gain2 : Gain  Gain=-1
  Product : Product
  Scope : Scope  NumInputPorts=2
  Sum : Sum  Inputs=|+-
  Sum1 : Sum  Inputs=|++
  Sum2 : Sum  Inputs=|+-
  Sum3 : Sum  Inputs=|++
  DutyOut : Outport
  wires:
  Constant/1 -> Sum1/2, Sum/2
  Product/1 -> Sum2/1, Sum/1
  Constant8/1 -> Divide2/2
  Constant7/1 -> Divide2/1
  Divide2/1 -> Divide/2
  Constant1/1 -> Divide/1
  Divide/1 -> Display/1, Product/1
  DutyIn/1 -> Product/2
  Gain1/1 -> Sum1/1
  Sum/1 -> Gain1/1
  Sum2/1 -> Dead Zone/1
  Gain2/1 -> Sum3/1
  Dead Zone/1 -> Gain2/1
  Constant2/1 -> Sum3/2, Sum2/2
  Sum3/1 -> DutyOut/1, Scope/1
  Sum1/1 -> Scope/2

== system Senorless/Subsystem2 ==
  Trigger : TriggerPort  TriggerType=function-call  VariantControl=(inherit)  PortDimensions=1
  Constant16 : Constant  Value=SPD_MAX  OutDataTypeStr=int16
  Product2 : Product
  Random Number1 : RandomNumber  Mean=0.5  Variance=0.0001  Seed=15
  Saturation1 : Saturate  UpperLimit=1  LowerLimit=0
  Out1 : Outport
  wires:
  Saturation1/1 -> Product2/1
  Constant16/1 -> Product2/2
  Random Number1/1 -> Saturation1/1
  Product2/1 -> Out1/1

== system Senorless/FOC_PointModel/AntiPark ==
  note: Valpha = ud*cos(theta) - uq*sin(theta);
      | Vbeta = ud*sin(theta) + uq*cos(theta);
  Ud : Inport
  Uq : Inport  Port=2
  Theta_Sin : Inport  Port=3
  Theta_Cos : Inport  Port=4
  Add : Sum  Inputs=+-  OutDataTypeStr=int32
  Add1 : Sum  OutDataTypeStr=int32
  Product{,1..3} (4 alike) : Product  OutDataTypeStr=int32  RndMeth=Zero
  Shift Arithmetic : ArithShift  BitShiftNumber=15  DiagnosticForOORShift=Error
  Shift Arithmetic1 : ArithShift  BitShiftNumber=15  DiagnosticForOORShift=Error
  Theta_Cos1 : InportShadow  Port=4
  Theta_Sin1 : InportShadow  Port=3
  Ud1 : InportShadow
  Uq1 : InportShadow  Port=2
  ualpha : Outport
  ubeta : Outport  Port=2
  wires:
  Theta_Cos/1 -> Product/2
  Ud/1 -> Product/1
  Add/1 -> Shift Arithmetic/1
  Shift Arithmetic/1 -> ualpha/1
  Shift Arithmetic1/1 -> ubeta/1
  Product1/1 -> Add/2
  Product/1 -> Add/1
  Uq/1 -> Product1/1
  Theta_Sin/1 -> Product1/2
  Add1/1 -> Shift Arithmetic1/1
  Product2/1 -> Add1/1
  Product3/1 -> Add1/2
  Ud1/1 -> Product2/1
  Theta_Sin1/1 -> Product2/2
  Theta_Cos1/1 -> Product3/2
  Uq1/1 -> Product3/1

== system Senorless/FOC_PointModel/Clark ==
  note: ialpha = ia;
      | ibeta = (ib-ic)/sqrt(3);
  ia : Inport
  ib : Inport  Port=2
  ic : Inport  Port=3
  Add2 : Sum  Inputs=+-  OutDataTypeStr=int32  RndMeth=Zero
  Gain2 : Gain  Gain=32767/sqrt(3)  ParamDataTypeStr=int16  OutDataTypeStr=int32  RndMeth=Zero
  Shift Arithmetic : ArithShift  BitShiftNumber=15  DiagnosticForOORShift=Error
  ialpha : Outport
  ibeta : Outport  Port=2
  wires:
  Gain2/1 -> Shift Arithmetic/1
  Add2/1 -> Gain2/1
  ic/1 -> Add2/2
  ib/1 -> Add2/1
  Shift Arithmetic/1 -> ibeta/1
  ia/1 -> ialpha/1

== system Senorless/FOC_PointModel/Err ==
  ia : Inport
  ib : Inport  Port=2
  ic : Inport  Port=3
  Obs_SPD : Inport  Port=4
  Udc_Ref : Inport  Port=5
  Reset : Inport  Port=6
  Abs1 : Abs  RndMeth=Zero  SaturateOnIntegerOverflow=off
  Abs2 : Abs  RndMeth=Zero  SaturateOnIntegerOverflow=off
  Abs3 : Abs  RndMeth=Zero  SaturateOnIntegerOverflow=off
  Data Store Read3 : DataStoreRead  DataStoreName=Curr_Over  IndexOptions=Index vector (dialog)  Indices=1  OutputSizes=1
  Max : MinMax  Function=max  Inputs=3  RndMeth=Zero
  PLL_LPF1 : Subsystem  TreatAsAtomicUnit=on
  Relational Operator : RelationalOperator  Operator=<  OutDataTypeStr=boolean  RndMeth=Zero  InputSameDT=off
  Relational Operator1 : RelationalOperator  Operator===  OutDataTypeStr=boolean  RndMeth=Zero  InputSameDT=off
  Scope : Scope
  Unit Delay : UnitDelay  SampleTime=-1  HasFrameUpgradeWarning=on
  闭环是4 : Constant  Value=4  OutDataTypeStr=uint8
  闭环错误判断 : Subsystem
  Over_Curr_Err : Outport
  Run_Err : Outport  Port=2
  wires:
  Abs2/1 -> Max/2
  Abs3/1 -> Max/3
  Data Store Read3/1 -> Relational Operator/1
  PLL_LPF1/1(output) -> Scope/1, 闭环错误判断/2(Curr_Max), Relational Operator/2
  Abs1/1 -> Max/1
  Max/1 -> PLL_LPF1/1(input)
  Relational Operator/1 -> 闭环错误判断/1(Curr_Err), Over_Curr_Err/1
  ic/1 -> Abs3/1
  ia/1 -> Abs1/1
  ib/1 -> Abs2/1
  Obs_SPD/1 -> 闭环错误判断/3(Obs_SPD)
  Udc_Ref/1 -> 闭环错误判断/4(Udc_Ref)
  闭环错误判断/1(Run_Err) -> Run_Err/1
  闭环是4/1 -> Relational Operator1/2
  Relational Operator1/1 -> 闭环错误判断/Enable
  Reset/1 -> Unit Delay/1
  Unit Delay/1 -> Relational Operator1/1

== system Senorless/FOC_PointModel/Observers ==
  note: 非线性磁链手脚架
  note: 观测器开发手脚架，包含浮点SMO、PLL，逐步定点化等步骤
  ualpha : Inport
  ialpha : Inport  Port=2
  ubeta : Inport  Port=3
  ibeta : Inport  Port=4
  Udc_Ref : Inport  Port=5
  Enable : EnablePort  StatesWhenEnabling=reset
  NFO : Subsystem  Commented=on
  PLL : Subsystem  TreatAsAtomicUnit=on
  PLL2 : Subsystem  Commented=on  TreatAsAtomicUnit=on
  SMO : Subsystem  TreatAsAtomicUnit=on
  Subsystem : Subsystem  Commented=on
  atan_1 : MATLAB Function  Commented=on  TreatAsAtomicUnit=on
  ialpha{1..4} (4 alike) : InportShadow  Port=2
  ibeta{1..4} (4 alike) : InportShadow  Port=4
  ualpha{1..4} (4 alike) : InportShadow
  ubeta{1..4} (4 alike) : InportShadow  Port=3
  浮点但是数量级是定点的NFO : Subsystem  Commented=on
  纯浮点NFO : Subsystem  Commented=on
  Obs_Spd : Outport
  Obs_Theta : Outport  Port=2
  wires:
  ualpha1/1 -> Subsystem/3(ualpha)
  ialpha1/1 -> Subsystem/6(ialpha)
  ubeta1/1 -> Subsystem/7(In7)
  ibeta1/1 -> Subsystem/8(In8)
  ialpha/1 -> SMO/2(ialpha)
  ibeta/1 -> SMO/4(ibeta)
  SMO/1(Ealpha) -> PLL/1(sin)
  ubeta/1 -> SMO/3(ubeta)
  ualpha/1 -> SMO/1(ualpha)
  ualpha3/1 -> 纯浮点NFO/1(ualpha)
  ialpha3/1 -> 纯浮点NFO/2(ialpha)
  ubeta3/1 -> 纯浮点NFO/3(ubeta)
  ibeta3/1 -> 纯浮点NFO/4(ibeta)
  ualpha2/1 -> 浮点但是数量级是定点的NFO/1(ualpha)
  ialpha2/1 -> 浮点但是数量级是定点的NFO/2(ialpha)
  ubeta2/1 -> 浮点但是数量级是定点的NFO/3(ubeta)
  ibeta2/1 -> 浮点但是数量级是定点的NFO/4(ibeta)
  ualpha4/1 -> NFO/1(ualpha)
  ialpha4/1 -> NFO/2(ialpha)
  ubeta4/1 -> NFO/3(ubeta)
  ibeta4/1 -> NFO/4(ibeta)
  Udc_Ref/1 -> NFO/5(Udc_Ref)
  SMO/2(Ebeta) -> PLL/2(cos)
  NFO/1(cos) -> PLL2/1(cos)
  NFO/2(sin) -> PLL2/2(sin)
  PLL/2(Obs_Theta) -> Obs_Theta/1
  PLL/1(Obs_Spd) -> Obs_Spd/1

== system Senorless/FOC_PointModel/Park ==
  note: id = ialpha*cos(theta)+ibeta*sin(theta);
      | iq = -ialpha*sin(theta)+ibeta*cos(theta);
  ialpha : Inport
  ibeta : Inport  Port=2
  Theta_Sin : Inport  Port=3
  Theta_Cos : Inport  Port=4
  Add1 : Sum  Inputs=-+
  Add2 : Sum
  Product{,1..3} (4 alike) : Product  OutDataTypeStr=int32  RndMeth=Zero
  Shift Arithmetic : ArithShift  BitShiftNumber=15  DiagnosticForOORShift=Error
  Shift Arithmetic1 : ArithShift  BitShiftNumber=15  DiagnosticForOORShift=Error
  Theta_Cos1 : InportShadow  Port=4
  Theta_Sin1 : InportShadow  Port=3
  ialpha1 : InportShadow
  ibeta1 : InportShadow  Port=2
  Id : Outport
  Iq : Outport  Port=2
  wires:
  Product1/1 -> Add2/2
  Add1/1 -> Shift Arithmetic1/1
  Add2/1 -> Shift Arithmetic/1
  Product/1 -> Add2/1
  Shift Arithmetic/1 -> Id/1
  ialpha/1 -> Product/1
  Theta_Cos/1 -> Product/2
  ibeta/1 -> Product1/1
  Theta_Sin/1 -> Product1/2
  ialpha1/1 -> Product2/1
  Theta_Sin1/1 -> Product2/2
  ibeta1/1 -> Product3/1
  Theta_Cos1/1 -> Product3/2
  Product2/1 -> Add1/1
  Product3/1 -> Add1/2
  Shift Arithmetic1/1 -> Iq/1

== system Senorless/FOC_PointModel/SVPWM ==
  note: 此处上下本应都乘一个Udc的，因为有相除所以可以约去
  Ualpha : Inport
  Ubeta : Inport  Port=2
  ia : Inport  Port=3
  ib : Inport  Port=4
  ic : Inport  Port=5
  AntiClark : Subsystem
  Data Store Read1 : DataStoreRead  Commented=on  DataStoreName=Uout_Max  IndexOptions=Index vector (dialog)  Indices=1  OutputSizes=1
  Data Store Read3 : DataStoreRead  DataStoreName=PWM_TH  IndexOptions=Index vector (dialog)  Indices=1  OutputSizes=1
  Data Store Read4 : DataStoreRead  DataStoreName=PWM_TH  IndexOptions=Index vector (dialog)  Indices=1  OutputSizes=1
  Data Type Conversion : DataTypeConversion  OutDataTypeStr=uint16  SaturateOnIntegerOverflow=off  RndMeth=Floor
  Divide : Product  Commented=on  Inputs=*/  OutDataTypeStr=int32  RndMeth=Zero
  Gain1 : Gain  Gain=-85  ParamDataTypeStr=int16  OutDataTypeStr=int32  RndMeth=Zero
  Mux : Mux  Inputs=3
  Mux1 : Mux  Inputs=3
  Product : Product  OutDataTypeStr=int32  RndMeth=Zero
  Scope : Scope  NumInputPorts=2
  Scope1 : Scope  NumInputPorts=2
  Shift Arithmetic : ArithShift  BitShiftNumber=1  DiagnosticForOORShift=Error
  Sign : Signum
  Sum : Sum  Inputs=++-  OutDataTypeStr=int32  RndMeth=Zero
  Sum1 : Sum  Inputs=++|  OutDataTypeStr=int16
  Unary Minus : UnaryMinus
  ei_t : Subsystem
  默认除以32767 : ArithShift  BitShiftNumber=15
  tABC : Outport
  wires:
  Ualpha/1 -> AntiClark/1(Valpha)
  Ubeta/1 -> AntiClark/2(Vbeta)
  ei_t/1(ei_t) -> Sum/1
  AntiClark/1(Va) -> Mux/1
  AntiClark/2(Vb) -> Mux/2
  AntiClark/3(Vc) -> Mux/3
  Mux/1 -> ei_t/1(Vabc), Sum/2
  Data Type Conversion/1 -> tABC/1, Scope/1
  Unary Minus/1 -> Sum1/2
  Sum1/1 -> Scope/2, Data Type Conversion/1
  Data Store Read3/1 -> Shift Arithmetic/1
  Shift Arithmetic/1 -> Sum1/1
  Product/1 -> 默认除以32767/1
  默认除以32767/1 -> Unary Minus/1
  Sum/1 -> Product/1, Scope1/2, Scope1/1
  ia/1 -> Mux1/1
  ib/1 -> Mux1/2
  ic/1 -> Mux1/3
  Mux1/1 -> Sign/1
  Sign/1 -> Gain1/1
  Data Store Read4/1 -> Product/2
  Gain1/1 -> Sum/3
